simulink model "perfIndx_th"  (R2018b)
settings: Solver=VariableStepAuto  StartTime=0.0  StopTime=0  RelTol=1e-3
values from neighbouring files (symbols this model uses):
  D = DBdyTrue    [fit6DoFDoF_ts1.m]    (also in perfIndx.m = rotMat * D; perfIndx_ts.m = [d1(:) d2(:) d3(:) d4(:)]; perfIndx_ts1.m = [d1(:) d2(:) d3(:) d4(:)])
  eulAngs = [0 0 45]    [perfIndx_ts.m]
  posVec = [0 0 50]    [perfIndx_ts.m]
  R = [r1(:) r2(:) r3(:) r4(:)]    [perfIndx_ts.m]    (also in perfIndx_ts1.m)
  U = [u1(:) u2(:) u3(:) u4(:)]    [perfIndx_ts.m]    (also in perfIndx_ts1.m)
  w = ones([1 numDots])    [fit6DoFDoF_ts1.m]    (also in perfIndx_ts.m = [1 1 1 1]; perfIndx_ts1.m = [1 1 1 1]; perfIndx_ts2.m)
settings Model: Creator=mcobb  LastModifiedBy=mcobb

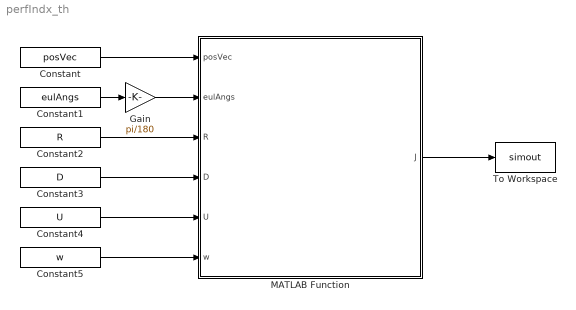
== system perfIndx_th ==
  Constant : Constant  Value=posVec
  Constant1 : Constant  Value=eulAngs
  Constant2 : Constant  Value=R
  Constant3 : Constant  Value=D
  Constant4 : Constant  Value=U
  Constant5 : Constant  Value=w
  Gain : Gain  Gain=pi/180
  MATLAB Function : MATLAB Function  TreatAsAtomicUnit=on
  To Workspace : ToWorkspace  VariableName=simout  SaveFormat=Timeseries  SampleTime=-1
  wires:
  Constant/1 -> MATLAB Function/1(posVec)
  MATLAB Function/1(J) -> To Workspace/1
  Constant1/1 -> Gain/1
  Gain/1 -> MATLAB Function/2(eulAngs)
  Constant2/1 -> MATLAB Function/3(R)
  Constant3/1 -> MATLAB Function/4(D)
  Constant4/1 -> MATLAB Function/5(U)
  Constant5/1 -> MATLAB Function/6(w)

== matlab function perfIndx_th/MATLAB Function ==
  data: posVec input; J output; eulAngs input; R input; D input; U input; w input
function J = fcn(posVec,eulAngs,R,D,U,w)

J = perfIndx(posVec,eulAngs,R,D,U,w);

end
